simulink model "Lorenza"  (R2022a)
settings: Solver=FixedStepAuto  StartTime=0.0  StopTime=25  FixedStep=0.001  RelTol=1e-3
settings Model: Creator=Tymon  LastModifiedBy=tymon
settings DebuggingCC: UnconnectedInputMsg=warning  UnconnectedOutputMsg=warning  UnconnectedLineMsg=warning
settings RTWCC: DLArmComputeVersion=19.05

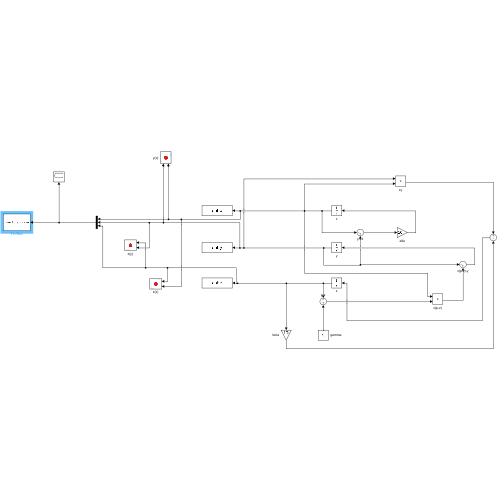
[thumbnail: Simulink's stored preview of the top-level diagram]
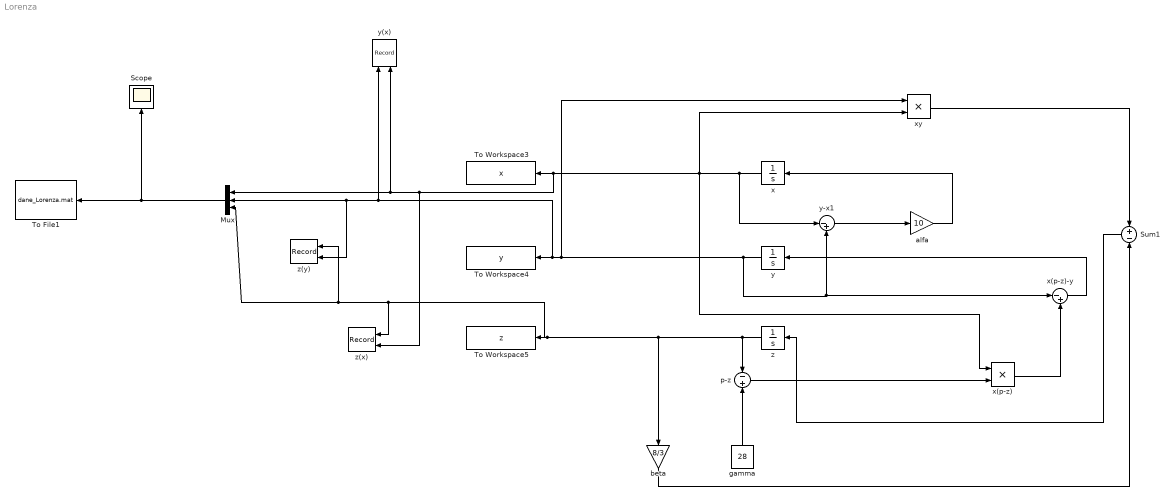
== system Lorenza ==
  Mux : Mux  Inputs=3
  Scope : Scope
  Sum1 : Sum  Inputs=+-
  To File1 : ToFile  Filename=dane_Lorenza.mat  MatrixName=dane_Lorenza
  To Workspace3 : ToWorkspace  VariableName=x  SampleTime=-1
  To Workspace4 : ToWorkspace  VariableName=y  SampleTime=-1
  To Workspace5 : ToWorkspace  VariableName=z  SampleTime=-1
  alfa : Gain  Gain=10
  beta : Gain  Gain=8/3
  gamma : Constant  Value=28
  p-z : Sum  Inputs=-+
  x : Integrator  InitialCondition=1
  x(p-z) : Product
  x(p-z)-y : Sum  Inputs=|-+
  xy : Product
  y : Integrator  InitialCondition=1
  y(x) : Record  FileSettingsInternal="{\"entries\":[{\"content\":{\"excelSettings\":{\"content\":{},\"type\":\"Streamout.ExcelSettings\"}},\"type\":\"Streamout.FileSettingStorage\",\"uuid\":\"f0942b12-394a-4738-83b7-571fd7ef9a39\"}],\"packageUris\":[\"http://schema.mathworks.com/mf0/streamout_blocks/R2020a\"],\"version\":\"1.0\"}"  Layout=[1 1]  SignalsInternal="{\"entries\":[{\"content\":{\"signals\":[{\"content\":{\"blockPath\":[\"Lorenza/y(x)\"],\"channel\":[],\"dimensions\":[1],\"domain\":\"Lorenza/y(x)\",\"lineColor\":\"#b746ff\",\"plots\":[1],\"port\":1,\"sid\":[\"\"],\"signalID\":654,\"signalName\":\"y\"},\"type\":\"RecordBlkView.Signal\",\"uuid\":\"7f44048a-cff7-4dd3-858b-5316345a4519\"},{\"content\":{\"blockPath\":[\"Lorenza/y(x)\"],\"channel\":[],\"dimensions\":[1],\"domain\":\"Lorenza/y(x)\",\"lineColor\":\"#b746ff\",\"plots\":[1],\"port\":2,\"sid\":[\"\"],\"signalID\":658,\"signalName\":\"x\"},\"type\":\"RecordBlkView.Signal\",\"uuid\":\"32227cf1-7f32-4ce2-9ea1-0d1f52f264ca\"}]},\"type\":\"RecordBlkView.InputSignals\",\"uuid\":\"fc7fb111-394b-4854-8c5e-27d7157d6285\"}],\"packageUris\":[\"http://schema.mathworks.com/mf0/streamout_blocks/R2020a\"],\"version\":\"1.0\"}"  VisualizationBindings="{\"xyplotplugin\":{\"info\":[{\"series\":[{\"bindingParametersList\":[{\"parameter\":\"Y-Axis\",\"signalID\":658,\"signalName\":\"x\"},{\"parameter\":\"X-Axis\",\"signalID\":654,\"signalName\":\"y\"}],\"seriesID\":57853}],\"subplotID\":1}]}}"  CompatibilityTag=XY
  y-x1 : Sum  Inputs=|-+
  z : Integrator  InitialCondition=1
  z(x) : Record  FileSettingsInternal="{\"entries\":[{\"content\":{\"excelSettings\":{\"content\":{},\"type\":\"Streamout.ExcelSettings\"}},\"type\":\"Streamout.FileSettingStorage\",\"uuid\":\"b4aea132-a40d-4a6b-983a-b2e098c8d11c\"}],\"packageUris\":[\"http://schema.mathworks.com/mf0/streamout_blocks/R2020a\"],\"version\":\"1.0\"}"  Layout=[1 1]  SignalsInternal="{\"entries\":[{\"content\":{\"signals\":[{\"content\":{\"blockPath\":[\"Lorenza/z(x)\"],\"channel\":[],\"dimensions\":[1],\"domain\":\"Lorenza/z(x)\",\"lineColor\":\"#ff13a6\",\"plots\":[1],\"port\":1,\"sid\":[\"\"],\"signalID\":662,\"signalName\":\"z\"},\"type\":\"RecordBlkView.Signal\",\"uuid\":\"66935d00-bb17-47a4-9bdd-c1d51e5b32b8\"},{\"content\":{\"blockPath\":[\"Lorenza/z(x)\"],\"channel\":[],\"dimensions\":[1],\"domain\":\"Lorenza/z(x)\",\"lineColor\":\"#fe330a\",\"plots\":[1],\"port\":2,\"sid\":[\"\"],\"signalID\":666,\"signalName\":\"x\"},\"type\":\"RecordBlkView.Signal\",\"uuid\":\"9fe805f4-d742-4522-b3e4-ca6122be48f1\"}]},\"type\":\"RecordBlkView.InputSignals\",\"uuid\":\"7ce8d526-7382-4ed2-8e3b-28ad27e74159\"}],\"packageUris\":[\"http://schema.mathworks.com/mf0/streamout_blocks/R2020a\"],\"version\":\"1.0\"}"  VisualizationBindings="{\"xyplotplugin\":{\"info\":[{\"series\":[{\"bindingParametersList\":[{\"parameter\":\"Y-Axis\",\"signalID\":662,\"signalName\":\"z\"},{\"parameter\":\"X-Axis\",\"signalID\":666,\"signalName\":\"x\"}],\"seriesID\":15199}],\"subplotID\":1}]}}"  CompatibilityTag=XY
  z(y) : Record  FileSettingsInternal="{\"entries\":[{\"content\":{\"excelSettings\":{\"content\":{},\"type\":\"Streamout.ExcelSettings\"}},\"type\":\"Streamout.FileSettingStorage\",\"uuid\":\"c5e5b71f-1c43-4f47-acd1-d058877d64a6\"}],\"packageUris\":[\"http://schema.mathworks.com/mf0/streamout_blocks/R2020a\"],\"version\":\"1.0\"}"  Layout=[1 1]  SignalsInternal="{\"entries\":[{\"content\":{\"signals\":[{\"content\":{\"blockPath\":[\"Lorenza/z(y)\"],\"channel\":[],\"dimensions\":[1],\"domain\":\"Lorenza/z(y)\",\"lineColor\":\"#22b573\",\"plots\":[1],\"port\":1,\"sid\":[\"\"],\"signalID\":670,\"signalName\":\"z\"},\"type\":\"RecordBlkView.Signal\",\"uuid\":\"5ded4605-2993-4b2e-aee9-fbf282f7f341\"},{\"content\":{\"blockPath\":[\"Lorenza/z(y)\"],\"channel\":[],\"dimensions\":[1],\"domain\":\"Lorenza/z(y)\",\"lineColor\":\"#0072bd\",\"plots\":[1],\"port\":2,\"sid\":[\"\"],\"signalID\":674,\"signalName\":\"y\"},\"type\":\"RecordBlkView.Signal\",\"uuid\":\"6ef9b9e9-ecfd-4914-af15-dc3ba40580ed\"}]},\"type\":\"RecordBlkView.InputSignals\",\"uuid\":\"254187fa-9bc9-4b92-aacd-ba1de7b0e5e2\"}],\"packageUris\":[\"http://schema.mathworks.com/mf0/streamout_blocks/R2020a\"],\"version\":\"1.0\"}"  VisualizationBindings="{\"xyplotplugin\":{\"info\":[{\"series\":[{\"bindingParametersList\":[{\"parameter\":\"Y-Axis\",\"signalID\":674,\"signalName\":\"y\"},{\"parameter\":\"X-Axis\",\"signalID\":670,\"signalName\":\"z\"}],\"seriesID\":54388}],\"subplotID\":1}]}}"  CompatibilityTag=XY
  wires:
  x/1 -> y-x1/1, xy/2, x(p-z)/1, z(x)/2, y(x)/2, Mux/1, To Workspace3/1
  y/1 -> xy/1, y(x)/1, z(y)/2, Mux/2, To Workspace4/1, y-x1/2, x(p-z)-y/1
  z/1 -> beta/1, z(x)/1, z(y)/1, Mux/3, To Workspace5/1, p-z/1
  y-x1/1 -> alfa/1
  alfa/1 -> x/1
  gamma/1 -> p-z/2
  p-z/1 -> x(p-z)/2
  x(p-z)/1 -> x(p-z)-y/2
  x(p-z)-y/1 -> y/1
  beta/1 -> Sum1/2
  xy/1 -> Sum1/1
  Sum1/1 -> z/1
  Mux/1 -> Scope/1, To File1/1
